simulink model "d01_Diaglnteg"  (R2024a)
settings: Solver=FixedStepDiscrete  StartTime=0.0  StopTime=1  FixedStep=mSim.dTime  MaxStep=Define.sModelSampleTime  RelTol=7.1420e-05
undefined symbols (not defined in the file): CnstMde, D01CRT, D01SPD, D01TEMP, D01VDC, D02DFLT
settings Model: Creator=user  LastModifiedBy=admin
settings SolverCC: MaxConsecutiveZCs=10000  ZeroCrossAlgorithm=Adaptive  AlgebraicLoopSolver=TrustRegion
settings DataIOCC: SaveOutput=off  DSMLogging=off  InspectSignalLogs=on  SaveTime=off  SignalLoggingName=logsout_Validator
settings OptimizationCC: BlockReduction=off  DefaultParameterBehavior=Inlined  UseDivisionForNetSlopeComputation=UseDivisionForReciprocalsOfIntegersOnly  GainParamInheritBuiltInType=on  UseFloatMulNetSlope=on  DefaultUnderspecifiedDataType=single  InlineInvariantSignals=on  BitwiseOrLogicalOp=Logical operator  PassReuseOutputArgsAs=Individual arguments  EfficientFloat2IntCast=on  LifeSpan=Inf  OptimizeBlockOrder=speed  DifferentSizesBufferReuse=on  EfficientTunableParamExpr=on
settings DebuggingCC: SignalInfNanChecking=error  SignalRangeChecking=error  ReadBeforeWriteMsg=EnableAllAsError  WriteAfterWriteMsg=EnableAllAsError  WriteAfterReadMsg=EnableAllAsError  AlgebraicLoopMsg=error  ArtificialAlgebraicLoopMsg=error  SaveWithDisabledLinksMsg=error  SaveWithParameterizedLinksMsg=error  BlockPriorityViolationMsg=error  SolverPrmCheckMsg=error  InheritedTsInSrcMsg=error  SingleTaskRateTransMsg=error  TasksWithSamePriorityMsg=error  SigSpecEnsureSampleTimeMsg=error  CheckMatrixSingularityMsg=error  IntegerOverflowMsg=error  ParameterUnderflowMsg=error  ParameterPrecisionLossMsg=error  ParameterTunabilityLossMsg=error  UnderSpecifiedDataTypeMsg=error  UnnecessaryDatatypeConvMsg=warning  VectorMatrixConversionMsg=error  SignalLabelMismatchMsg=error  UnconnectedInputMsg=error  UnconnectedOutputMsg=error  UnconnectedLineMsg=error  SFcnCompatibilityMsg=error  UniqueDataStoreMsg=error  BusObjectLabelMismatch=error  RootOutportRequireBusObject=error  AssertControl=DisableAll  ModelReferenceIOMismatchMessage=error  UnknownTsInhSupMsg=error  ModelReferenceDataLoggingMessage=error  ModelReferenceSymbolNameMessage=none  StateNameClashWarn=warning  StrictBusMsg=ErrorOnBusTreatedAsVector  NonBusSignalsTreatedAsBus=error  SFInvalidInputDataAccessInChartInitDiag=error  SFTransitionOutsideNaturalParentDiag=error  SFUnreachableExecutionPathDiag=error  SFUndirectedBroadcastEventsDiag=error  SFTransitionActionBeforeConditionDiag=error  SFTemporalDelaySmallerThanSampleTimeDiag=error  SFSelfTransitionDiag=error  SFExecutionAtInitializationDiag=error  IntegerSaturationMsg=error  UnitsInconsistencyMsg=none  VariantConditionMismatch=error
settings HardwareCC: ProdBitPerChar=16  ProdBitPerInt=16  ProdBitPerPointer=32  ProdBitPerSizeT=32  ProdBitPerPtrDiffT=32  ProdLargestAtomicInteger=Integer  ProdLargestAtomicFloat=None  ProdWordSize=16  ProdHWDeviceType=Texas Instruments->C2000
settings ModelReferenceCC: EnableRefExpFcnMdlSchedulingChecks=on  ModelReferenceNumInstancesAllowed=Single
settings SFSimCC: SimUseLocalCustomCode=off  CompileTimeRecursionLimit=0  EnableRuntimeRecursion=off  MATLABDynamicMemAlloc=off  CustomCodeUndefinedFunction=UseInterfaceOnly
settings RTWCC: Description=Embedded Coder  SystemTargetFile=ert.tlc  GenCodeOnly=on  TemplateMakefile=ert_default_tmf  GenerateReport=on  RTWUseLocalCustomCode=off  BuildConfiguration=Faster Runs  IncludeHyperlinkInReport=on  LaunchReport=on  GenerateTraceInfo=on  GenerateTraceReport=on  GenerateTraceReportSl=on  GenerateTraceReportSf=on  GenerateWebview=on  GenerateCodeMetricsReport=on  GenerateCodeReplacementReport=on  GPUComputeCapability=3.5  DLArmComputeVersion=19.05
settings CodeAppCC: ForceParamTrailComments=on  IgnoreCustomStorageClasses=off  MATLABFcnDesc=on  MangleLength=4  CustomSymbolStrGlobalVar=GvD01$N$M  CustomSymbolStrType=StrD01$N$M  CustomSymbolStrFcn=$N$M$F  CustomSymbolStrMacro=$N$M  DefineNamingRule=UpperCase  ParamNamingRule=UpperCase  SimulinkBlockComments=off  MATLABSourceComments=on  EnableCustomComments=on  ReqsInCode=on
settings ERTTargetCC: TargetLangStandard=C99 (ISO)  UtilityFuncGeneration=Shared location  MultiwordLength=2048  IncludeMdlTerminateFcn=off  CombineSignalStateStructs=on  SuppressErrorStatus=on  SupportAbsoluteTime=off  SupportNonFinite=off  ParenthesesLevel=Maximum  CastingMode=Standards  GenerateSharedConstants=off  InlinedParameterPlacement=NonHierarchical  ERTSrcFileBannerTemplate=t_code_template.cgt  ERTHdrFileBannerTemplate=t_code_template.cgt  ERTDataSrcFileTemplate=t_code_template.cgt  ERTDataHdrFileTemplate=t_code_template.cgt  ERTCustomFileTemplate=example_file_process.tlc  ERTFilePackagingFormat=CompactWithDataFile  PreserveExpressionOrder=on  SuppressUnreachableDefaultCases=off  EnableSignedLeftShifts=off  EnableSignedRightShifts=off  IndentStyle=Allman  IndentSize=4
settings ConfigComp: CovSaveName=coveragedata  CovMetricSettings=we  CovEnableCumulative=off  CovSaveCumulativeToWorkspaceVar=on  CovSaveSingleToWorkspaceVar=on  CovOutputDir=sldv_output/$ModelName$\sldv_covoutput  PSVerificationMode=BugFinder  PSModelRefIgnoreList=[]  PSEnableModelRefIgnoreList=off  PSModelRefMinMaxVerif=CheckAndConstrain  PSAutoStubLUT=on  DVModelCoverageObjectives=MCDC  DVTestSuiteOptimization=CombinedObjectives (Nonlinear Extended)  DVRebuildModelRepresentation=Always
settings SimscapeCC: SimscapeNormalizeSystem=off

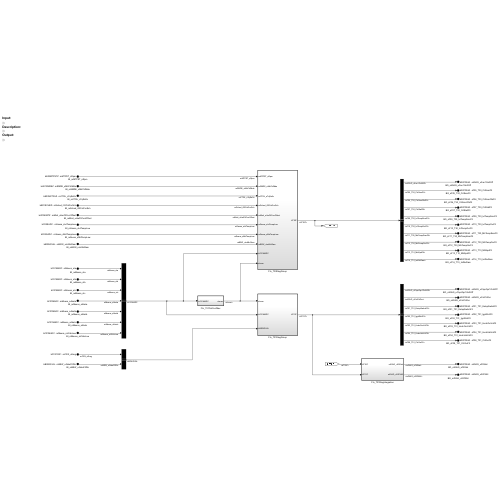
[thumbnail: Simulink's stored preview of the top-level diagram]
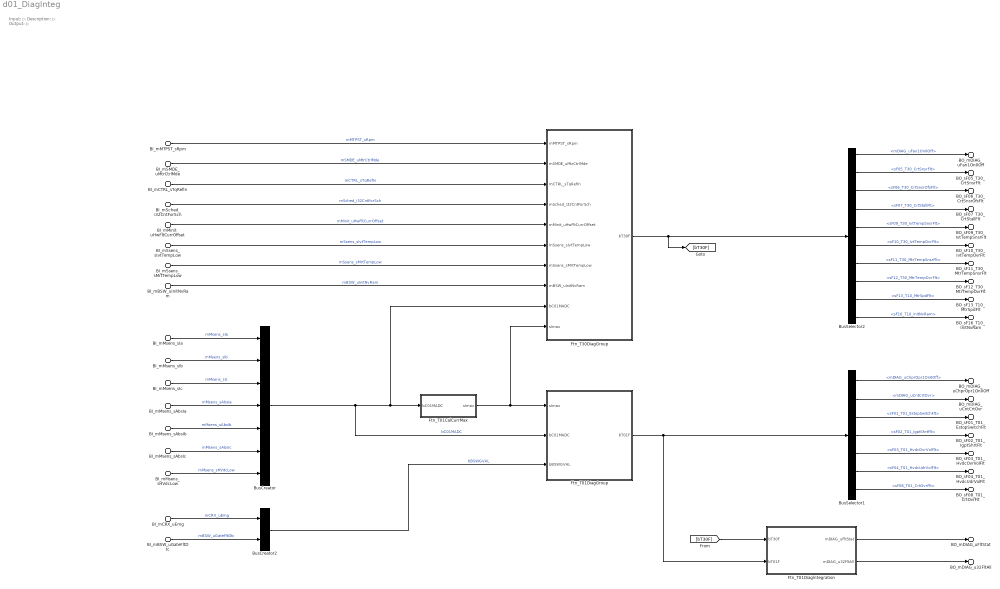
== system d01_Diaglnteg ==
  note: Input:
      | ▷
      | Description:
      | ▷
      | Output:
      | ▷
  BI_mMsens_sIa : Inport  PortName=bC01MADC  Element=mMsens_sIa
  BI_mMsens_sIb : Inport  PortName=bC01MADC  Element=mMsens_sIb
  BI_mMsens_sIc : Inport  PortName=bC01MADC  Element=mMsens_sIc
  BI_mMsens_sAbsIa : Inport  PortName=bC01MADC  Element=mMsens_sAbsIa
  BI_mMsens_sAbsIb : Inport  PortName=bC01MADC  Element=mMsens_sAbsIb
  BI_mMsens_sAbsIc : Inport  PortName=bC01MADC  Element=mMsens_sAbsIc
  BI_mMsens_sHVdcLow : Inport  PortName=bC01MADC  Element=mMsens_sHVdcLow
  BI_mSched_i32CntForSch : Inport  Port=2  PortName=bB01SCHED  Element=mSched_i32CntForSch
  BI_mMinit_uHwFltCurrOffset : Inport  Port=3  PortName=bJ01MINITZ  Element=mMinit_uHwFltCurrOffset
  BI_mCTRL_sTqRefIn : Inport  Port=4  PortName=bE03MCTRLZ  Element=mCTRL_sTqRefIn
  BI_mBSW_uGateFltDtc : Inport  Port=5  PortName=bBSWGVAL  Element=mBSW_uGateFltDtc
  BI_mBSW_uInitNvRam : Inport  Port=5  PortName=bBSWGVAL  Element=mBSW_uInitNvRam
  BI_mMTPST_sRpm : Inport  Port=6  PortName=bE02MTPSTZ  Element=mMTPST_sRpm
  BI_mSsens_sIvtTempLow : Inport  Port=7  PortName=bC02SADC  Element=mSsens_sIvtTempLow
  BI_mSsens_sMrtTempLow : Inport  Port=7  PortName=bC02SADC  Element=mSsens_sMrtTempLow
  BI_mSMDE_uMtrCtrlMde : Inport  Port=8  PortName=bH01SMDEZ  Element=mSMDE_uMtrCtrlMde
  BI_mCRX_uEmg : Inport  Description=■ 설명: Digital Input Signal (외부 비상 신호 입력, 0: 비상 신호 활성화, 1: 비상 신호 비활성화)  Port=9  PortName=bF01CRX1  Element=mCRX_uEmg
  BusCreator : BusCreator  Inputs=7
  BusCreator2 : BusCreator  Inputs=2
  BusSelector1 : BusSelector  OutputSignals=mDIAG_uChprOpr1On0Off,mDIAG_uCntCrtOvr,sF01_T01_EstopSwitchFlt,sF02_T01_IgptShrtFlt,sF03_T01_HvdcOvrVolFlt,sF04_T01_HvdcUdrVolFlt,sF08_T01_CrtOvrFlt
  BusSelector2 : BusSelector  OutputSignals=mDIAG_uFan1On0Off,sF05_T30_CrtSnsrFlt,sF06_T30_CrtSnsrOfsFlt,sF07_T30_CrtStallFlt,sF09_T30_IvtTempSnsrFlt,sF10_T30_IvtTempOvrFlt,sF11_T30_MtrTempSnsrFlt,sF12_T30_MtrTempOvrFlt,sF13_T10_MtrSpdFlt,sF16_T10_InitNvRam
  Ftn_T01CalCurrMax : Subsystem  TreatAsAtomicUnit=on
      settings: RTWSystemCode=Nonreusable function  RTWFcnNameOpts=Use subsystem name
  Ftn_T01DiagGroup : Subsystem  TreatAsAtomicUnit=on
      settings: RTWSystemCode=Nonreusable function  RTWFcnNameOpts=Use subsystem name
  Ftn_T01Diaglntegration : Subsystem  TreatAsAtomicUnit=on
      settings: RTWSystemCode=Nonreusable function  RTWFcnNameOpts=Use subsystem name
  Ftn_T30DiagGroup : Subsystem  TreatAsAtomicUnit=on
      settings: RTWSystemCode=Nonreusable function  RTWFcnNameOpts=Use subsystem name
  BO_mDIAG_uFltStat : Outport  Description=■ 설명: 고장 신호 대표 값  PortName=bD01DIAG  Element=mDIAG_uFltStat
  BO_mDIAG_u32FltAll : Outport  Description=■ 설명: 고장 신호 전체값  PortName=bD01DIAG  Element=mDIAG_u32FltAll
  BO_mDIAG_uChprOpr1On0Off : Outport  Description=■ 설명: Chopper 구동 신호 (0: Off, 1: On)  PortName=bD01DIAG  Element=mDIAG_uChprOpr1On0Off
  BO_mDIAG_uFan1On0Off : Outport  Description=■ 설명: Fan 구동 신호 (0: Off, 1: On)  PortName=bD01DIAG  Element=mDIAG_uFan1On0Off
  BO_mDIAG_uCntCrtOvr : Outport  Description=■ 설명: 과전류 검출 카운터  PortName=bD01DIAG  Element=mDIAG_uCntCrtOvr
  BO_sF01_T01_EstopSwitchFlt : Outport  Description=■ 설명: E-Stop Swhitch 검출 (0: Normal, 1: Fault)  PortName=bD01DIAG  Element=sF01_T01_EstopSwitchFlt
  BO_sF02_T01_IgptShrtFlt : Outport  Description=■ 설명: IGBT 고장 신호 (0: Normal, 1: Fault)  PortName=bD01DIAG  Element=sF02_T01_IgptShrtFlt
  BO_sF03_T01_HvdcOvrVolFlt : Outport  Description=■ 설명: DC Link 과전압 고장 검출 신호 (0: Normal, 1: Fault)  PortName=bD01DIAG  Element=sF03_T01_HvdcOvrVolFlt
  BO_sF04_T01_HvdcUdrVolFlt : Outport  Description=■ 설명: DC Link 저전압 고장 검출 신호 (0: Normal, 1: Fault)  PortName=bD01DIAG  Element=sF04_T01_HvdcUdrVolFlt
  BO_sF05_T30_CrtSnsrFlt : Outport  Description=■ 설명: 전류 센서 고장 검출 신호 (0: Normal, 1: Fault)  PortName=bD01DIAG  Element=sF05_T30_CrtSnsrFlt
  BO_sF06_T30_CrtSnsrOfsFlt : Outport  Description=■ 설명: 전류 센서 옵셋 고장 검출 신호 (0: Normal, 1: Fault)  PortName=bD01DIAG  Element=sF06_T30_CrtSnsrOfsFlt
  BO_sF07_T30_CrtStallFlt : Outport  Description=■ 설명: 구속 전류 고장 검출 신호 (0: Normal, 1: Fault)  PortName=bD01DIAG  Element=sF07_T30_CrtStallFlt
  BO_sF08_T01_CrtOvrFlt : Outport  Description=■ 설명: 과전류 고장 검출 신호 (0: Normal, 1: Fault)  PortName=bD01DIAG  Element=sF08_T01_CrtOvrFlt
  BO_sF09_T30_IvtTempSnsrFlt : Outport  Description=■ 설명: IGBT 온도 센서 고장 검출 신호 (0: Normal, 1: Fault)  PortName=bD01DIAG  Element=sF09_T30_IvtTempSnsrFlt
  BO_sF10_T30_IvtTempOvrFlt : Outport  Description=■ 설명: IGBT 과온 고장 검출 신호 (0: Normal, 1: Fault)  PortName=bD01DIAG  Element=sF10_T30_IvtTempOvrFlt
  BO_sF11_T30_MtrTempSnsrFlt : Outport  Description=■ 설명: 모터 온도 센서 고장 검출 신호 (0: Normal, 1: Fault)  PortName=bD01DIAG  Element=sF11_T30_MtrTempSnsrFlt
  BO_sF12_T30_MtrTempOvrFlt : Outport  Description=■ 설명: 모터 과온 고장 검출 신호 (0: Normal, 1: Fault)  PortName=bD01DIAG  Element=sF12_T30_MtrTempOvrFlt
  BO_sF13_T10_MtrSpdFlt : Outport  Description="■ 설명: 과속 고장 검출 신호  (0: Normal, 1: Fault)"  PortName=bD01DIAG  Element=sF13_T10_MtrSpdFlt
  BO_sF16_T10_InitNvRam : Outport  Description=■ 설명: 모터 과온 고장 검출 신호 (0: Normal, 1: Fault)  PortName=bD01DIAG  Element=sF16_T10_InitNvRam
  wires:
  BI_mMsens_sIa/1 -> BusCreator/1  "mMsens_sIa"
  BI_mMsens_sIb/1 -> BusCreator/2  "mMsens_sIb"
  BI_mMsens_sIc/1 -> BusCreator/3  "mMsens_sIc"
  BI_mMsens_sAbsIa/1 -> BusCreator/4  "mMsens_sAbsIa"
  BI_mMsens_sAbsIb/1 -> BusCreator/5  "mMsens_sAbsIb"
  BI_mMsens_sAbsIc/1 -> BusCreator/6  "mMsens_sAbsIc"
  BI_mMsens_sHVdcLow/1 -> BusCreator/7  "mMsens_sHVdcLow"
  BusCreator/1 -> Ftn_T01CalCurrMax/1(bC01MADC), Ftn_T30DiagGroup/9(bC01MADC), Ftn_T01DiagGroup/2(bC01MADC)  "bC01MADC"
  Ftn_T01CalCurrMax/1(sImax) -> Ftn_T30DiagGroup/10(sImax), Ftn_T01DiagGroup/1(sImax)
  Ftn_T01DiagGroup/1(bT01F) -> BusSelector1/1, Ftn_T01Diaglntegration/2(bT01F)
  BusSelector1/1 -> BO_mDIAG_uChprOpr1On0Off/1  "<mDIAG_uChprOpr1On0Off>"
  BusSelector1/5 -> BO_sF03_T01_HvdcOvrVolFlt/1  "<sF03_T01_HvdcOvrVolFlt>"
  BusSelector1/6 -> BO_sF04_T01_HvdcUdrVolFlt/1  "<sF04_T01_HvdcUdrVolFlt>"
  BI_mSched_i32CntForSch/1 -> Ftn_T30DiagGroup/4(mSched_i32CntForSch)  "mSched_i32CntForSch"
  BusSelector1/7 -> BO_sF08_T01_CrtOvrFlt/1  "<sF08_T01_CrtOvrFlt>"
  BusSelector1/2 -> BO_mDIAG_uCntCrtOvr/1  "<mDIAG_uCntCrtOvr>"
  BI_mMinit_uHwFltCurrOffset/1 -> Ftn_T30DiagGroup/5(mMinit_uHwFltCurrOffset)  "mMinit_uHwFltCurrOffset"
  BI_mSMDE_uMtrCtrlMde/1 -> Ftn_T30DiagGroup/2(mSMDE_uMtrCtrlMde)  "mSMDE_uMtrCtrlMde"
  BI_mCTRL_sTqRefIn/1 -> Ftn_T30DiagGroup/3(mCTRL_sTqRefIn)  "mCTRL_sTqRefIn"
  Ftn_T30DiagGroup/1(bT30F) -> [bT30F], BusSelector2/1
  BusSelector2/2 -> BO_sF05_T30_CrtSnsrFlt/1  "<sF05_T30_CrtSnsrFlt>"
  BusSelector2/3 -> BO_sF06_T30_CrtSnsrOfsFlt/1  "<sF06_T30_CrtSnsrOfsFlt>"
  BusSelector2/4 -> BO_sF07_T30_CrtStallFlt/1  "<sF07_T30_CrtStallFlt>"
  BI_mBSW_uGateFltDtc/1 -> BusCreator2/2  "mBSW_uGateFltDtc"
  BusCreator2/1 -> Ftn_T01DiagGroup/3(bBSWGVAL)  "bBSWGVAL"
  BusSelector1/3 -> BO_sF01_T01_EstopSwitchFlt/1  "<sF01_T01_EstopSwitchFlt>"
  BusSelector1/4 -> BO_sF02_T01_IgptShrtFlt/1  "<sF02_T01_IgptShrtFlt>"
  BI_mMTPST_sRpm/1 -> Ftn_T30DiagGroup/1(mMTPST_sRpm)  "mMTPST_sRpm"
  BusSelector2/9 -> BO_sF13_T10_MtrSpdFlt/1  "<sF13_T10_MtrSpdFlt>"
  BI_mSsens_sIvtTempLow/1 -> Ftn_T30DiagGroup/6(mSsens_sIvtTempLow)  "mSsens_sIvtTempLow"
  BI_mSsens_sMrtTempLow/1 -> Ftn_T30DiagGroup/7(mSsens_sMrtTempLow)  "mSsens_sMrtTempLow"
  BusSelector2/5 -> BO_sF09_T30_IvtTempSnsrFlt/1  "<sF09_T30_IvtTempSnsrFlt>"
  BusSelector2/6 -> BO_sF10_T30_IvtTempOvrFlt/1  "<sF10_T30_IvtTempOvrFlt>"
  BusSelector2/7 -> BO_sF11_T30_MtrTempSnsrFlt/1  "<sF11_T30_MtrTempSnsrFlt>"
  BusSelector2/8 -> BO_sF12_T30_MtrTempOvrFlt/1  "<sF12_T30_MtrTempOvrFlt>"
  BusSelector2/1 -> BO_mDIAG_uFan1On0Off/1  "<mDIAG_uFan1On0Off>"
  [bT30F] -> Ftn_T01Diaglntegration/1(bT30F)
  Ftn_T01Diaglntegration/2(mDIAG_u32FltAll) -> BO_mDIAG_u32FltAll/1
  Ftn_T01Diaglntegration/1(mDIAG_uFltStat) -> BO_mDIAG_uFltStat/1
  BI_mBSW_uInitNvRam/1 -> Ftn_T30DiagGroup/8(mBSW_uInitNvRam)  "mBSW_uInitNvRam"
  BusSelector2/10 -> BO_sF16_T10_InitNvRam/1  "<sF16_T10_InitNvRam>"
  BI_mCRX_uEmg/1 -> BusCreator2/1  "mCRX_uEmg"

== system d01_Diaglnteg/Ftn_T01CalCurrMax ==
  note: Input:
      | Description:
      | Output:
  bC01MADC : Inport
  BusSelector : BusSelector  OutputSignals=mMsens_sAbsIa,mMsens_sAbsIb,mMsens_sAbsIc
  Max : MinMax  Function=max  Inputs=3
  sImax : Outport
  wires:
  Max/1 -> sImax/1  "sImax"
  bC01MADC/1 -> BusSelector/1
  BusSelector/2 -> Max/2  "<mMsens_sAbsIb>"
  BusSelector/1 -> Max/1  "<mMsens_sAbsIa>"
  BusSelector/3 -> Max/3  "<mMsens_sAbsIc>"

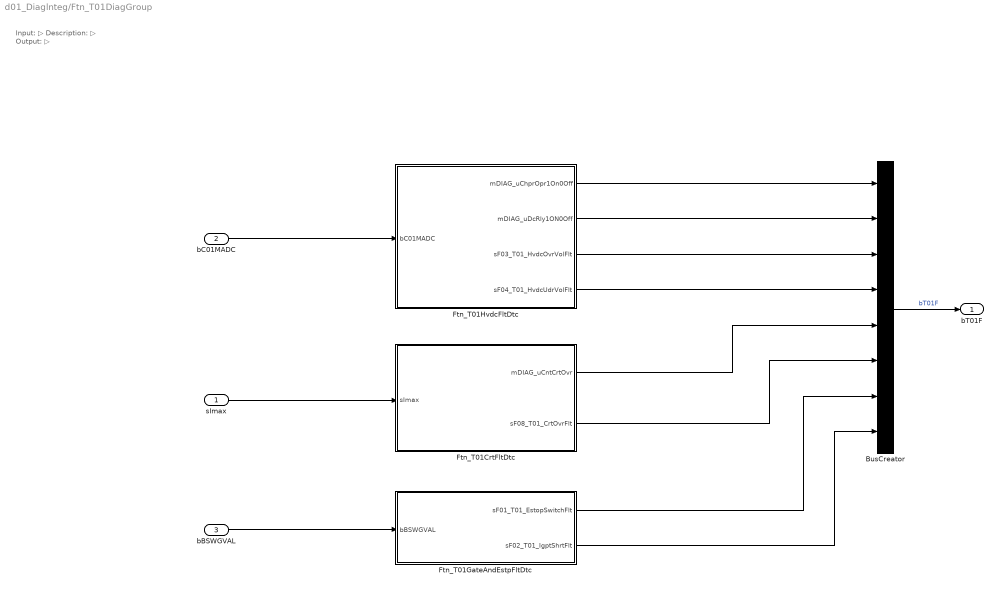
== system d01_Diaglnteg/Ftn_T01DiagGroup ==
  note: Input:
      | ▷
      | Description:
      | ▷
      | Output:
      | ▷
  sImax : Inport
  bC01MADC : Inport  Port=2
  bBSWGVAL : Inport  Port=3
  BusCreator : BusCreator  Inputs=8
  Ftn_T01CrtFltDtc : Subsystem  TreatAsAtomicUnit=on
      settings: RTWSystemCode=Nonreusable function  RTWFcnNameOpts=Use subsystem name
  Ftn_T01GateAndEstpFltDtc : Subsystem  TreatAsAtomicUnit=on
      settings: RTWSystemCode=Nonreusable function  RTWFcnNameOpts=Use subsystem name
  Ftn_T01HvdcFltDtc : Subsystem  TreatAsAtomicUnit=on
      settings: RTWSystemCode=Nonreusable function  RTWFcnNameOpts=Use subsystem name
  bT01F : Outport
  wires:
  bC01MADC/1 -> Ftn_T01HvdcFltDtc/1(bC01MADC)
  sImax/1 -> Ftn_T01CrtFltDtc/1(sImax)
  Ftn_T01HvdcFltDtc/1(mDIAG_uChprOpr1On0Off) -> BusCreator/1
  Ftn_T01HvdcFltDtc/3(sF03_T01_HvdcOvrVolFlt) -> BusCreator/3
  Ftn_T01HvdcFltDtc/4(sF04_T01_HvdcUdrVolFlt) -> BusCreator/4
  BusCreator/1 -> bT01F/1  "bT01F"
  Ftn_T01CrtFltDtc/1(mDIAG_uCntCrtOvr) -> BusCreator/5
  Ftn_T01CrtFltDtc/2(sF08_T01_CrtOvrFlt) -> BusCreator/6
  Ftn_T01GateAndEstpFltDtc/1(sF01_T01_EstopSwitchFlt) -> BusCreator/7
  bBSWGVAL/1 -> Ftn_T01GateAndEstpFltDtc/1(bBSWGVAL)
  Ftn_T01GateAndEstpFltDtc/2(sF02_T01_IgptShrtFlt) -> BusCreator/8
  Ftn_T01HvdcFltDtc/2(mDIAG_uDcRly1ON0Off) -> BusCreator/2

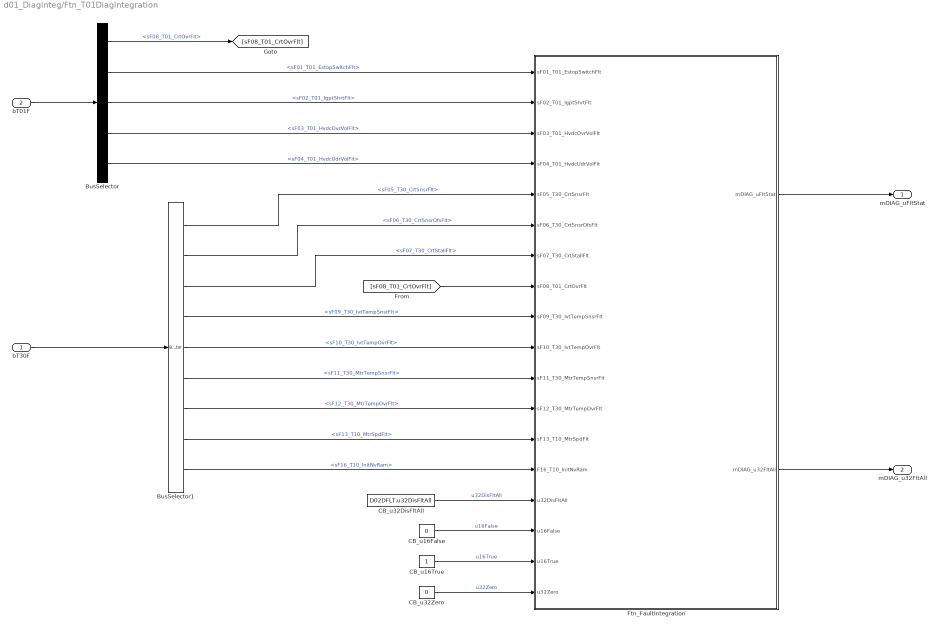
== system d01_Diaglnteg/Ftn_T01Diaglntegration ==
  bT30F : Inport
  bT01F : Inport  Port=2
  BusSelector : BusSelector  OutputSignals=sF08_T01_CrtOvrFlt,sF01_T01_EstopSwitchFlt,sF02_T01_IgptShrtFlt,sF03_T01_HvdcOvrVolFlt,sF04_T01_HvdcUdrVolFlt
  BusSelector1 : BusSelector  OutputSignals=sF05_T30_CrtSnsrFlt,sF06_T30_CrtSnsrOfsFlt,sF07_T30_CrtStallFlt,sF09_T30_IvtTempSnsrFlt,sF10_T30_IvtTempOvrFlt,sF11_T30_MtrTempSnsrFlt,sF12_T30_MtrTempOvrFlt,sF13_T10_MtrSpdFlt,sF16_T10_InitNvRam
  CB_u16False : Constant  Value=0  OutDataTypeStr=uint16
  CB_u16True : Constant  OutDataTypeStr=uint16
  CB_u32DisFltAll : Constant  Value=D02DFLT.u32DisFltAll
  CB_u32Zero : Constant  Value=0  OutDataTypeStr=uint32
  Ftn_FaultIntegration : Stateflow chart  TreatAsAtomicUnit=on
      settings: RTWSystemCode=Nonreusable function
  mDIAG_uFltStat : Outport
  mDIAG_u32FltAll : Outport  Port=2
  wires:
  bT01F/1 -> BusSelector/1
  BusSelector/2 -> Ftn_FaultIntegration/1(sF01_T01_EstopSwitchFlt)  "<sF01_T01_EstopSwitchFlt>"
  BusSelector/3 -> Ftn_FaultIntegration/2(sF02_T01_IgptShrtFlt)  "<sF02_T01_IgptShrtFlt>"
  BusSelector/1 -> [sF08_T01_CrtOvrFlt]  "<sF08_T01_CrtOvrFlt>"
  bT30F/1 -> BusSelector1/1
  BusSelector1/2 -> Ftn_FaultIntegration/6(sF06_T30_CrtSnsrOfsFlt)  "<sF06_T30_CrtSnsrOfsFlt>"
  BusSelector1/3 -> Ftn_FaultIntegration/7(sF07_T30_CrtStallFlt)  "<sF07_T30_CrtStallFlt>"
  BusSelector1/4 -> Ftn_FaultIntegration/9(sF09_T30_IvtTempSnsrFlt)  "<sF09_T30_IvtTempSnsrFlt>"
  BusSelector1/5 -> Ftn_FaultIntegration/10(sF10_T30_IvtTempOvrFlt)  "<sF10_T30_IvtTempOvrFlt>"
  BusSelector1/6 -> Ftn_FaultIntegration/11(sF11_T30_MtrTempSnsrFlt)  "<sF11_T30_MtrTempSnsrFlt>"
  BusSelector1/7 -> Ftn_FaultIntegration/12(sF12_T30_MtrTempOvrFlt)  "<sF12_T30_MtrTempOvrFlt>"
  BusSelector1/8 -> Ftn_FaultIntegration/13(sF13_T10_MtrSpdFlt)  "<sF13_T10_MtrSpdFlt>"
  BusSelector/4 -> Ftn_FaultIntegration/3(sF03_T01_HvdcOvrVolFlt)  "<sF03_T01_HvdcOvrVolFlt>"
  BusSelector/5 -> Ftn_FaultIntegration/4(sF04_T01_HvdcUdrVolFlt)  "<sF04_T01_HvdcUdrVolFlt>"
  BusSelector1/1 -> Ftn_FaultIntegration/5(sF05_T30_CrtSnsrFlt)  "<sF05_T30_CrtSnsrFlt>"
  [sF08_T01_CrtOvrFlt] -> Ftn_FaultIntegration/8(sF08_T01_CrtOvrFlt)
  CB_u32DisFltAll/1 -> Ftn_FaultIntegration/15(u32DisFltAll)  "u32DisFltAll"
  CB_u16False/1 -> Ftn_FaultIntegration/16(u16False)  "u16False"
  CB_u16True/1 -> Ftn_FaultIntegration/17(u16True)  "u16True"
  CB_u32Zero/1 -> Ftn_FaultIntegration/18(u32Zero)  "u32Zero"
  Ftn_FaultIntegration/1(mDIAG_uFltStat) -> mDIAG_uFltStat/1
  Ftn_FaultIntegration/2(mDIAG_u32FltAll) -> mDIAG_u32FltAll/1
  BusSelector1/9 -> Ftn_FaultIntegration/14(F16_T10_InitNvRam)  "<sF16_T10_InitNvRam>"

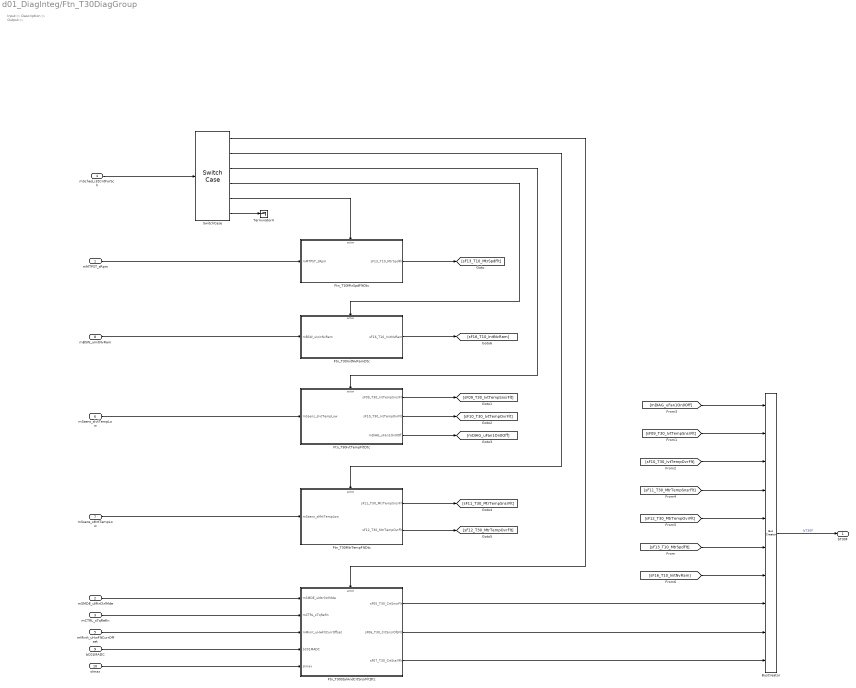
== system d01_Diaglnteg/Ftn_T30DiagGroup ==
  note: Input:
      | ▷
      | Description:
      | ▷
      | Output:
      | ▷
  mMTPST_sRpm : Inport
  mSMDE_uMtrCtrlMde : Inport  Port=2
  mCTRL_sTqRefIn : Inport  Port=3
  mSched_i32CntForSch : Inport  Port=4
  mMinit_uHwFltCurrOffset : Inport  Port=5
  mSsens_sIvtTempLow : Inport  Port=6
  mSsens_sMrtTempLow : Inport  Port=7
  mBSW_uInitNvRam : Inport  Port=8
  bC01MADC : Inport  Port=9
  sImax : Inport  Port=10
  BusCreator : BusCreator  Inputs=10
  Ftn_T10MtrSpdFltDtc : Subsystem  TreatAsAtomicUnit=on
      settings: RTWSystemCode=Nonreusable function  RTWFcnNameOpts=Use subsystem name
  Ftn_T30InitNvRamDtc : Subsystem
      settings: RTWSystemCode=Nonreusable function  RTWFcnNameOpts=Use subsystem name
  Ftn_T30IvtTempFltDtc : Subsystem  TreatAsAtomicUnit=on
      settings: RTWSystemCode=Nonreusable function  RTWFcnNameOpts=Use subsystem name
  Ftn_T30MtrTempFltDtc : Subsystem  TreatAsAtomicUnit=on
      settings: RTWSystemCode=Nonreusable function  RTWFcnNameOpts=Use subsystem name
  Ftn_T30StalAndCrtSnsrFltDtc : Subsystem  TreatAsAtomicUnit=on
      settings: RTWSystemCode=Nonreusable function  RTWFcnNameOpts=Use subsystem name
  SwitchCase : SwitchCase  CaseConditions={28, 24,18, 2, [6,26]}
  Terminator4 : Terminator
  bT30F : Outport
  wires:
  SwitchCase/6 -> Terminator4/1
  mSched_i32CntForSch/1 -> SwitchCase/1
  mMinit_uHwFltCurrOffset/1 -> Ftn_T30StalAndCrtSnsrFltDtc/3(mMinit_uHwFltCurrOffset)
  bC01MADC/1 -> Ftn_T30StalAndCrtSnsrFltDtc/4(bC01MADC)
  sImax/1 -> Ftn_T30StalAndCrtSnsrFltDtc/5(sImax)
  mCTRL_sTqRefIn/1 -> Ftn_T30StalAndCrtSnsrFltDtc/2(mCTRL_sTqRefIn)
  mSMDE_uMtrCtrlMde/1 -> Ftn_T30StalAndCrtSnsrFltDtc/1(mSMDE_uMtrCtrlMde)
  Ftn_T30StalAndCrtSnsrFltDtc/1(sF05_T30_CrtSnsrFlt) -> BusCreator/8
  Ftn_T30StalAndCrtSnsrFltDtc/2(sF06_T30_CrtSnsrOfsFlt) -> BusCreator/9
  Ftn_T30StalAndCrtSnsrFltDtc/3(sF07_T30_CrtStallFlt) -> BusCreator/10
  BusCreator/1 -> bT30F/1  "bT30F"
  SwitchCase/1 -> Ftn_T30StalAndCrtSnsrFltDtc/Action
  SwitchCase/4 -> Ftn_T30InitNvRamDtc/Action
  mMTPST_sRpm/1 -> Ftn_T10MtrSpdFltDtc/1(mMTPST_sRpm)
  Ftn_T10MtrSpdFltDtc/1(sF13_T10_MtrSpdFlt) -> [sF13_T10_MtrSpdFlt]
  [sF13_T10_MtrSpdFlt] -> BusCreator/6
  SwitchCase/3 -> Ftn_T30IvtTempFltDtc/Action
  mSsens_sIvtTempLow/1 -> Ftn_T30IvtTempFltDtc/1(mSsens_sIvtTempLow)
  Ftn_T30IvtTempFltDtc/1(sF09_T30_IvtTempSnsrFlt) -> [sF09_T30_IvtTempSnsrFlt]
  Ftn_T30IvtTempFltDtc/2(sF10_T30_IvtTempOvrFlt) -> [sF10_T30_IvtTempOvrFlt]
  Ftn_T30IvtTempFltDtc/3(mDIAG_uFan1On0Off) -> [mDIAG_uFan1On0Off]
  [sF09_T30_IvtTempSnsrFlt] -> BusCreator/2
  [sF10_T30_IvtTempOvrFlt] -> BusCreator/3
  [mDIAG_uFan1On0Off] -> BusCreator/1
  mSsens_sMrtTempLow/1 -> Ftn_T30MtrTempFltDtc/1(mSsens_sMrtTempLow)
  Ftn_T30MtrTempFltDtc/1(sF11_T30_MtrTempSnsrFlt) -> [sF11_T30_MtrTempSnsrFlt]
  Ftn_T30MtrTempFltDtc/2(sF12_T30_MtrTempOvrFlt) -> [sF12_T30_MtrTempOvrFlt]
  [sF11_T30_MtrTempSnsrFlt] -> BusCreator/4
  [sF12_T30_MtrTempOvrFlt] -> BusCreator/5
  SwitchCase/2 -> Ftn_T30MtrTempFltDtc/Action
  mBSW_uInitNvRam/1 -> Ftn_T30InitNvRamDtc/1(mBSW_uInitNvRam)
  Ftn_T30InitNvRamDtc/1(sF16_T10_InitNvRam) -> [sF16_T10_InitNvRam]
  [sF16_T10_InitNvRam] -> BusCreator/7
  SwitchCase/5 -> Ftn_T10MtrSpdFltDtc/Action

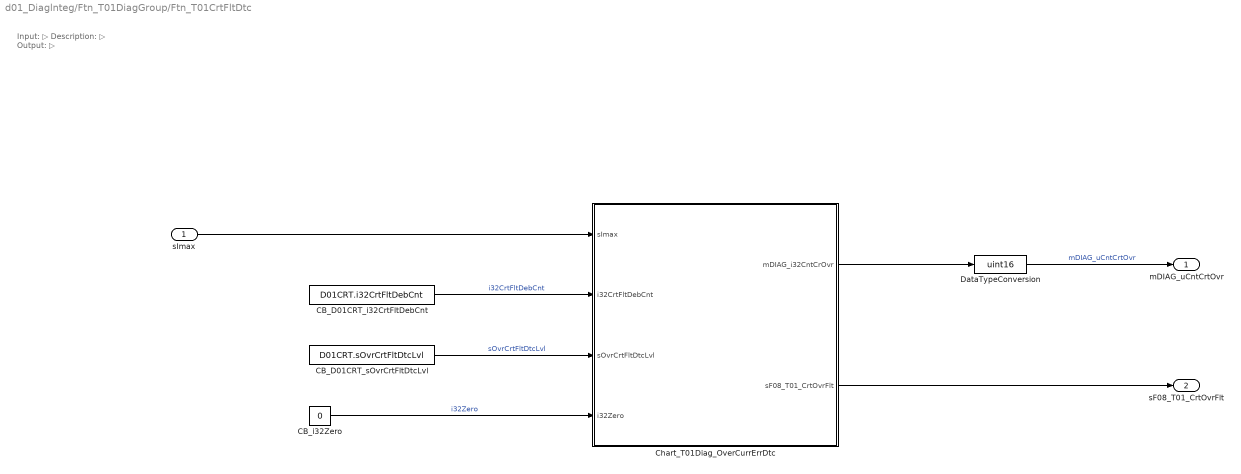
== system d01_Diaglnteg/Ftn_T01DiagGroup/Ftn_T01CrtFltDtc ==
  note: Input:
      | ▷
      | Description:
      | ▷
      | Output:
      | ▷
  sImax : Inport
  CB_D01CRT_i32CrtFltDebCnt : Constant  Value=D01CRT.i32CrtFltDebCnt
  CB_D01CRT_sOvrCrtFltDtcLvl : Constant  Value=D01CRT.sOvrCrtFltDtcLvl
  CB_i32Zero : Constant  Value=0  OutDataTypeStr=int32
  Chart_T01Diag_OverCurrErrDtc : Stateflow chart  TreatAsAtomicUnit=on
  DataTypeConversion : DataTypeConversion  OutDataTypeStr=uint16  SaturateOnIntegerOverflow=off  RndMeth=Floor
  mDIAG_uCntCrtOvr : Outport
  sF08_T01_CrtOvrFlt : Outport  Port=2
  wires:
  DataTypeConversion/1 -> mDIAG_uCntCrtOvr/1  "mDIAG_uCntCrtOvr"
  CB_i32Zero/1 -> Chart_T01Diag_OverCurrErrDtc/4(i32Zero)  "i32Zero"
  Chart_T01Diag_OverCurrErrDtc/1(mDIAG_i32CntCrOvr) -> DataTypeConversion/1
  Chart_T01Diag_OverCurrErrDtc/2(sF08_T01_CrtOvrFlt) -> sF08_T01_CrtOvrFlt/1
  CB_D01CRT_sOvrCrtFltDtcLvl/1 -> Chart_T01Diag_OverCurrErrDtc/3(sOvrCrtFltDtcLvl)  "sOvrCrtFltDtcLvl"
  CB_D01CRT_i32CrtFltDebCnt/1 -> Chart_T01Diag_OverCurrErrDtc/2(i32CrtFltDebCnt)  "i32CrtFltDebCnt"
  sImax/1 -> Chart_T01Diag_OverCurrErrDtc/1(sImax)

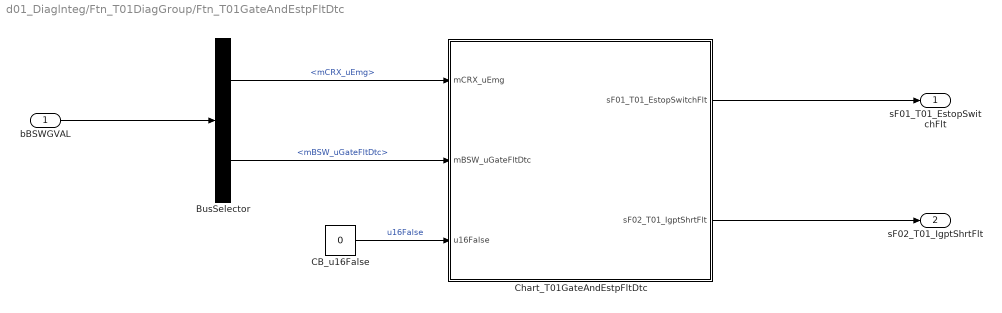
== system d01_Diaglnteg/Ftn_T01DiagGroup/Ftn_T01GateAndEstpFltDtc ==
  bBSWGVAL : Inport
  BusSelector : BusSelector  OutputSignals=mCRX_uEmg,mBSW_uGateFltDtc
  CB_u16False : Constant  Value=0  OutDataTypeStr=uint16
  Chart_T01GateAndEstpFltDtc : Stateflow chart  TreatAsAtomicUnit=on
  sF01_T01_EstopSwitchFlt : Outport
  sF02_T01_IgptShrtFlt : Outport  Port=2
  wires:
  bBSWGVAL/1 -> BusSelector/1
  BusSelector/1 -> Chart_T01GateAndEstpFltDtc/1(mCRX_uEmg)  "<mCRX_uEmg>"
  BusSelector/2 -> Chart_T01GateAndEstpFltDtc/2(mBSW_uGateFltDtc)  "<mBSW_uGateFltDtc>"
  Chart_T01GateAndEstpFltDtc/1(sF01_T01_EstopSwitchFlt) -> sF01_T01_EstopSwitchFlt/1
  Chart_T01GateAndEstpFltDtc/2(sF02_T01_IgptShrtFlt) -> sF02_T01_IgptShrtFlt/1
  CB_u16False/1 -> Chart_T01GateAndEstpFltDtc/3(u16False)  "u16False"

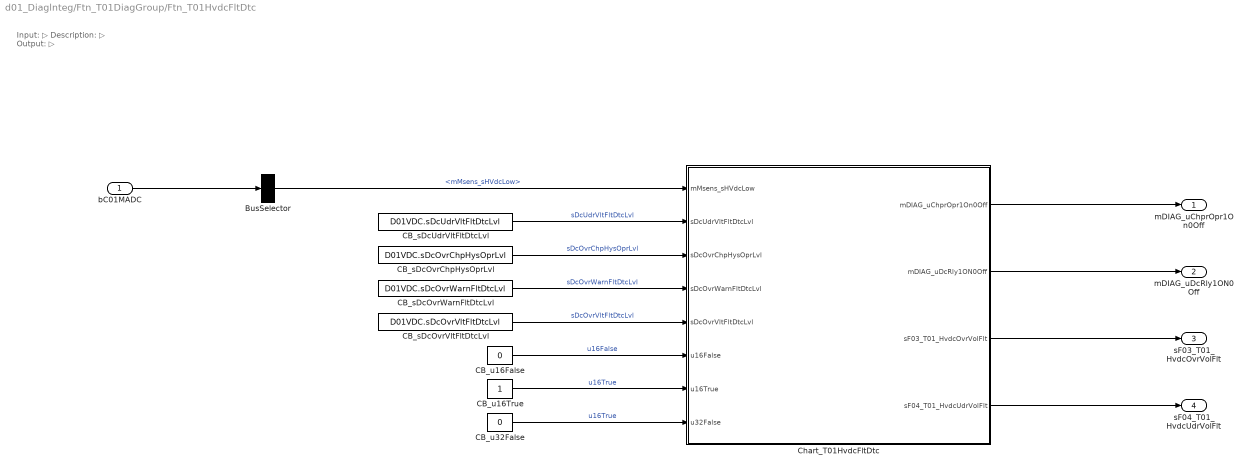
== system d01_Diaglnteg/Ftn_T01DiagGroup/Ftn_T01HvdcFltDtc ==
  note: Input:
      | ▷
      | Description:
      | ▷
      | Output:
      | ▷
  bC01MADC : Inport
  BusSelector : BusSelector  OutputSignals=mMsens_sHVdcLow
  CB_sDcOvrChpHysOprLvl : Constant  Value=D01VDC.sDcOvrChpHysOprLvl
  CB_sDcOvrVltFltDtcLvl : Constant  Value=D01VDC.sDcOvrVltFltDtcLvl
  CB_sDcOvrWarnFltDtcLvl : Constant  Value=D01VDC.sDcOvrWarnFltDtcLvl
  CB_sDcUdrVltFltDtcLvl : Constant  Value=D01VDC.sDcUdrVltFltDtcLvl
  CB_u16False : Constant  Value=0  OutDataTypeStr=uint16
  CB_u16True : Constant  OutDataTypeStr=uint16
  CB_u32False : Constant  Value=0  OutDataTypeStr=uint32
  Chart_T01HvdcFltDtc : Stateflow chart  TreatAsAtomicUnit=on
  mDIAG_uChprOpr1On0Off : Outport
  mDIAG_uDcRly1ON0Off : Outport  Port=2
  sF03_T01_HvdcOvrVolFlt : Outport  Port=3
  sF04_T01_HvdcUdrVolFlt : Outport  Port=4
  wires:
  bC01MADC/1 -> BusSelector/1
  BusSelector/1 -> Chart_T01HvdcFltDtc/1(mMsens_sHVdcLow)  "<mMsens_sHVdcLow>"
  CB_sDcUdrVltFltDtcLvl/1 -> Chart_T01HvdcFltDtc/2(sDcUdrVltFltDtcLvl)  "sDcUdrVltFltDtcLvl"
  CB_sDcOvrChpHysOprLvl/1 -> Chart_T01HvdcFltDtc/3(sDcOvrChpHysOprLvl)  "sDcOvrChpHysOprLvl"
  CB_sDcOvrWarnFltDtcLvl/1 -> Chart_T01HvdcFltDtc/4(sDcOvrWarnFltDtcLvl)  "sDcOvrWarnFltDtcLvl"
  CB_sDcOvrVltFltDtcLvl/1 -> Chart_T01HvdcFltDtc/5(sDcOvrVltFltDtcLvl)  "sDcOvrVltFltDtcLvl"
  CB_u16False/1 -> Chart_T01HvdcFltDtc/6(u16False)  "u16False"
  CB_u16True/1 -> Chart_T01HvdcFltDtc/7(u16True)  "u16True"
  Chart_T01HvdcFltDtc/1(mDIAG_uChprOpr1On0Off) -> mDIAG_uChprOpr1On0Off/1
  Chart_T01HvdcFltDtc/3(sF03_T01_HvdcOvrVolFlt) -> sF03_T01_HvdcOvrVolFlt/1
  Chart_T01HvdcFltDtc/4(sF04_T01_HvdcUdrVolFlt) -> sF04_T01_HvdcUdrVolFlt/1
  Chart_T01HvdcFltDtc/2(mDIAG_uDcRly1ON0Off) -> mDIAG_uDcRly1ON0Off/1
  CB_u32False/1 -> Chart_T01HvdcFltDtc/8(u32False)  "u16True"

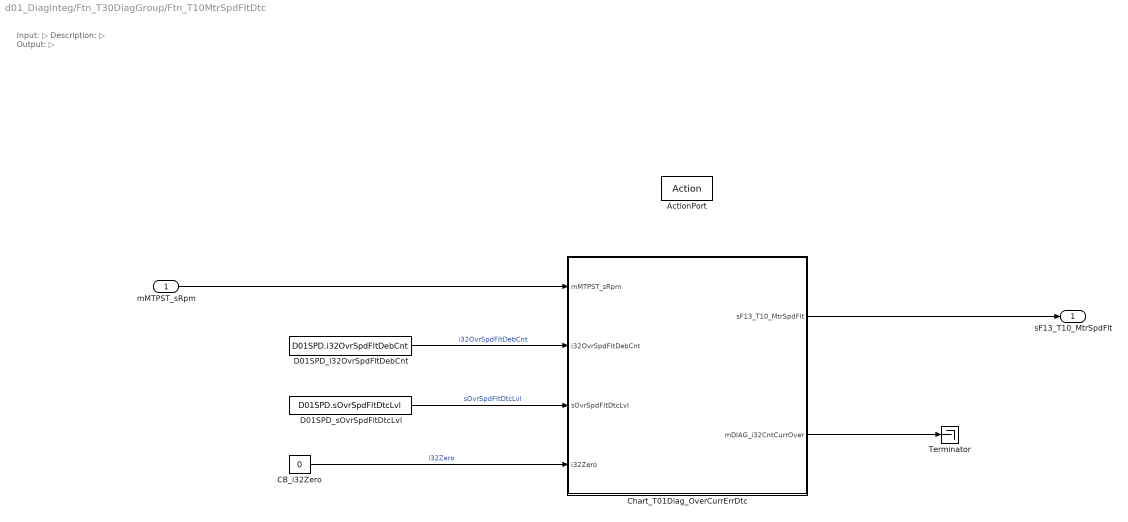
== system d01_Diaglnteg/Ftn_T30DiagGroup/Ftn_T10MtrSpdFltDtc ==
  note: Input:
      | ▷
      | Description:
      | ▷
      | Output:
      | ▷
  mMTPST_sRpm : Inport
  ActionPort : ActionPort  ActionPortLabel=case [ 6 26 ]:
  CB_i32Zero : Constant  Value=0  OutDataTypeStr=int32
  Chart_T01Diag_OverCurrErrDtc : Stateflow chart  TreatAsAtomicUnit=on
  D01SPD_i32OvrSpdFltDebCnt : Constant  Value=D01SPD.i32OvrSpdFltDebCnt
  D01SPD_sOvrSpdFltDtcLvl : Constant  Value=D01SPD.sOvrSpdFltDtcLvl
  Terminator : Terminator
  sF13_T10_MtrSpdFlt : Outport
  wires:
  D01SPD_sOvrSpdFltDtcLvl/1 -> Chart_T01Diag_OverCurrErrDtc/3(sOvrSpdFltDtcLvl)  "sOvrSpdFltDtcLvl"
  Chart_T01Diag_OverCurrErrDtc/1(sF13_T10_MtrSpdFlt) -> sF13_T10_MtrSpdFlt/1
  D01SPD_i32OvrSpdFltDebCnt/1 -> Chart_T01Diag_OverCurrErrDtc/2(i32OvrSpdFltDebCnt)  "i32OvrSpdFltDebCnt"
  CB_i32Zero/1 -> Chart_T01Diag_OverCurrErrDtc/4(i32Zero)  "i32Zero"
  Chart_T01Diag_OverCurrErrDtc/2(mDIAG_i32CntCurrOver) -> Terminator/1
  mMTPST_sRpm/1 -> Chart_T01Diag_OverCurrErrDtc/1(mMTPST_sRpm)

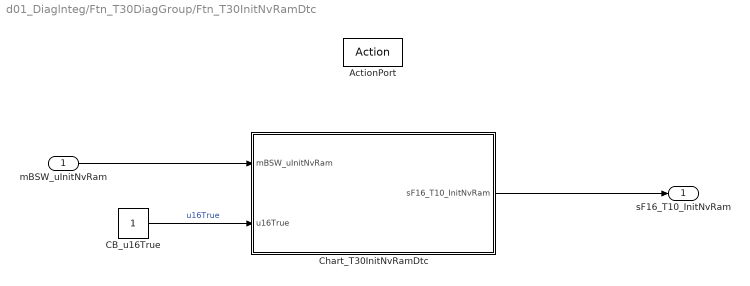
== system d01_Diaglnteg/Ftn_T30DiagGroup/Ftn_T30InitNvRamDtc ==
  mBSW_uInitNvRam : Inport
  ActionPort : ActionPort  ActionPortLabel=case [ 2 ]:
  CB_u16True : Constant  OutDataTypeStr=uint16
  Chart_T30InitNvRamDtc : Stateflow chart  TreatAsAtomicUnit=on
  sF16_T10_InitNvRam : Outport
  wires:
  CB_u16True/1 -> Chart_T30InitNvRamDtc/2(u16True)  "u16True"
  mBSW_uInitNvRam/1 -> Chart_T30InitNvRamDtc/1(mBSW_uInitNvRam)
  Chart_T30InitNvRamDtc/1(sF16_T10_InitNvRam) -> sF16_T10_InitNvRam/1

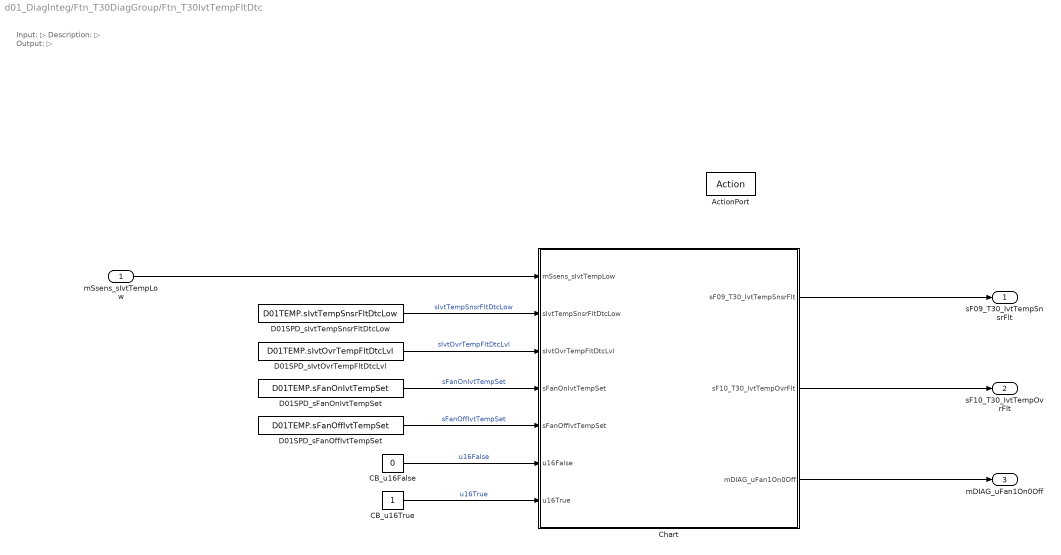
== system d01_Diaglnteg/Ftn_T30DiagGroup/Ftn_T30IvtTempFltDtc ==
  note: Input:
      | ▷
      | Description:
      | ▷
      | Output:
      | ▷
  mSsens_sIvtTempLow : Inport
  ActionPort : ActionPort  ActionPortLabel=case [ 18 ]:
  CB_u16False : Constant  Value=0  OutDataTypeStr=uint16
  CB_u16True : Constant  OutDataTypeStr=uint16
  Chart : Stateflow chart  TreatAsAtomicUnit=on
  D01SPD_sFanOffIvtTempSet : Constant  Value=D01TEMP.sFanOffIvtTempSet
  D01SPD_sFanOnIvtTempSet : Constant  Value=D01TEMP.sFanOnIvtTempSet
  D01SPD_sIvtOvrTempFltDtcLvl : Constant  Value=D01TEMP.sIvtOvrTempFltDtcLvl
  D01SPD_sIvtTempSnsrFltDtcLow : Constant  Value=D01TEMP.sIvtTempSnsrFltDtcLow
  sF09_T30_IvtTempSnsrFlt : Outport
  sF10_T30_IvtTempOvrFlt : Outport  Port=2
  mDIAG_uFan1On0Off : Outport  Port=3
  wires:
  mSsens_sIvtTempLow/1 -> Chart/1(mSsens_sIvtTempLow)
  Chart/1(sF09_T30_IvtTempSnsrFlt) -> sF09_T30_IvtTempSnsrFlt/1
  D01SPD_sIvtOvrTempFltDtcLvl/1 -> Chart/3(sIvtOvrTempFltDtcLvl)  "sIvtOvrTempFltDtcLvl"
  D01SPD_sFanOnIvtTempSet/1 -> Chart/4(sFanOnIvtTempSet)  "sFanOnIvtTempSet"
  D01SPD_sFanOffIvtTempSet/1 -> Chart/5(sFanOffIvtTempSet)  "sFanOffIvtTempSet"
  D01SPD_sIvtTempSnsrFltDtcLow/1 -> Chart/2(sIvtTempSnsrFltDtcLow)  "sIvtTempSnsrFltDtcLow"
  Chart/2(sF10_T30_IvtTempOvrFlt) -> sF10_T30_IvtTempOvrFlt/1
  CB_u16False/1 -> Chart/6(u16False)  "u16False"
  CB_u16True/1 -> Chart/7(u16True)  "u16True"
  Chart/3(mDIAG_uFan1On0Off) -> mDIAG_uFan1On0Off/1

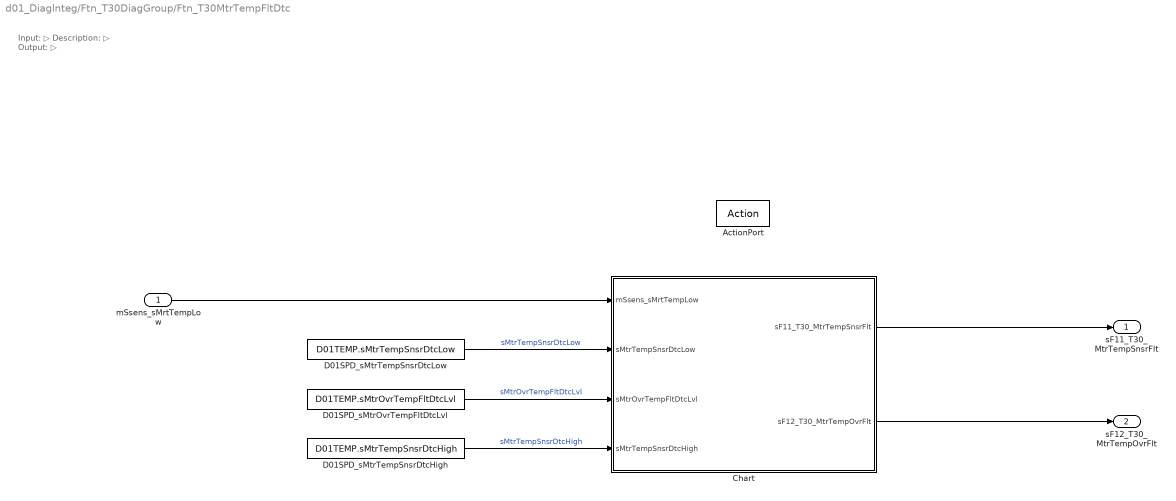
== system d01_Diaglnteg/Ftn_T30DiagGroup/Ftn_T30MtrTempFltDtc ==
  note: Input:
      | ▷
      | Description:
      | ▷
      | Output:
      | ▷
  mSsens_sMrtTempLow : Inport
  ActionPort : ActionPort  ActionPortLabel=case [ 24 ]:
  Chart : Stateflow chart  TreatAsAtomicUnit=on
  D01SPD_sMtrOvrTempFltDtcLvl : Constant  Value=D01TEMP.sMtrOvrTempFltDtcLvl
  D01SPD_sMtrTempSnsrDtcHigh : Constant  Value=D01TEMP.sMtrTempSnsrDtcHigh
  D01SPD_sMtrTempSnsrDtcLow : Constant  Value=D01TEMP.sMtrTempSnsrDtcLow
  sF11_T30_MtrTempSnsrFlt : Outport
  sF12_T30_MtrTempOvrFlt : Outport  Port=2
  wires:
  Chart/2(sF12_T30_MtrTempOvrFlt) -> sF12_T30_MtrTempOvrFlt/1
  D01SPD_sMtrTempSnsrDtcLow/1 -> Chart/2(sMtrTempSnsrDtcLow)  "sMtrTempSnsrDtcLow"
  D01SPD_sMtrTempSnsrDtcHigh/1 -> Chart/4(sMtrTempSnsrDtcHigh)  "sMtrTempSnsrDtcHigh"
  D01SPD_sMtrOvrTempFltDtcLvl/1 -> Chart/3(sMtrOvrTempFltDtcLvl)  "sMtrOvrTempFltDtcLvl"
  Chart/1(sF11_T30_MtrTempSnsrFlt) -> sF11_T30_MtrTempSnsrFlt/1
  mSsens_sMrtTempLow/1 -> Chart/1(mSsens_sMrtTempLow)

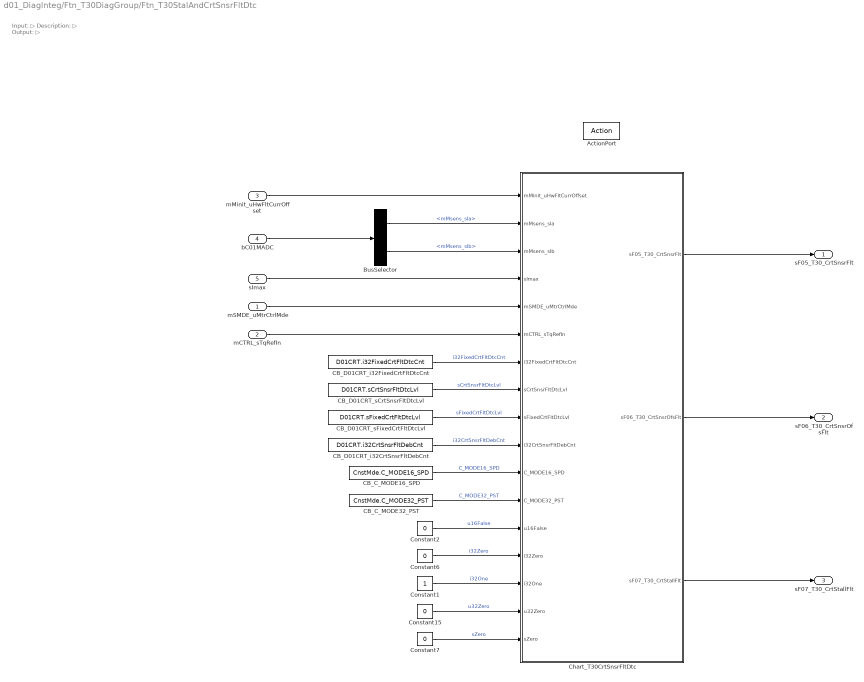
== system d01_Diaglnteg/Ftn_T30DiagGroup/Ftn_T30StalAndCrtSnsrFltDtc ==
  note: Input:
      | ▷
      | Description:
      | ▷
      | Output:
      | ▷
  mSMDE_uMtrCtrlMde : Inport
  mCTRL_sTqRefIn : Inport  Port=2
  mMinit_uHwFltCurrOffset : Inport  Port=3
  bC01MADC : Inport  Port=4
  sImax : Inport  Port=5  OutMin=0  OutMax=325.2
  ActionPort : ActionPort  ActionPortLabel=case [ 28 ]:
  BusSelector : BusSelector  OutputSignals=mMsens_sIa,mMsens_sIb
  CB_C_MODE16_SPD : Constant  Value=CnstMde.C_MODE16_SPD
  CB_C_MODE32_PST : Constant  Value=CnstMde.C_MODE32_PST
  CB_D01CRT_i32CrtSnsrFltDebCnt : Constant  Value=D01CRT.i32CrtSnsrFltDebCnt
  CB_D01CRT_i32FixedCrtFltDtcCnt : Constant  Value=D01CRT.i32FixedCrtFltDtcCnt
  CB_D01CRT_sCrtSnsrFltDtcLvl : Constant  Value=D01CRT.sCrtSnsrFltDtcLvl
  CB_D01CRT_sFixedCrtFltDtcLvl : Constant  Value=D01CRT.sFixedCrtFltDtcLvl
  Chart_T30CrtSnsrFltDtc : Stateflow chart  TreatAsAtomicUnit=on
  Constant1 : Constant  OutDataTypeStr=int32
  Constant15 : Constant  Value=0  OutDataTypeStr=uint32
  Constant2 : Constant  Value=0  OutDataTypeStr=uint16
  Constant6 : Constant  Value=0  OutDataTypeStr=int32
  Constant7 : Constant  Value=0  OutDataTypeStr=single
  sF05_T30_CrtSnsrFlt : Outport
  sF06_T30_CrtSnsrOfsFlt : Outport  Port=2  OutMin=0  OutMax=65536
  sF07_T30_CrtStallFlt : Outport  Port=3
  wires:
  CB_D01CRT_sCrtSnsrFltDtcLvl/1 -> Chart_T30CrtSnsrFltDtc/8(sCrtSnsrFltDtcLvl)  "sCrtSnsrFltDtcLvl"
  CB_D01CRT_i32FixedCrtFltDtcCnt/1 -> Chart_T30CrtSnsrFltDtc/7(i32FixedCrtFltDtcCnt)  "i32FixedCrtFltDtcCnt"
  sImax/1 -> Chart_T30CrtSnsrFltDtc/4(sImax)
  Constant15/1 -> Chart_T30CrtSnsrFltDtc/16(u32Zero)  "u32Zero"
  Constant1/1 -> Chart_T30CrtSnsrFltDtc/15(i32One)  "i32One"
  Chart_T30CrtSnsrFltDtc/2(sF06_T30_CrtSnsrOfsFlt) -> sF06_T30_CrtSnsrOfsFlt/1
  CB_D01CRT_i32CrtSnsrFltDebCnt/1 -> Chart_T30CrtSnsrFltDtc/10(i32CrtSnsrFltDebCnt)  "i32CrtSnsrFltDebCnt"
  Constant2/1 -> Chart_T30CrtSnsrFltDtc/13(u16False)  "u16False"
  Constant7/1 -> Chart_T30CrtSnsrFltDtc/17(sZero)  "sZero"
  Constant6/1 -> Chart_T30CrtSnsrFltDtc/14(i32Zero)  "i32Zero"
  mMinit_uHwFltCurrOffset/1 -> Chart_T30CrtSnsrFltDtc/1(mMinit_uHwFltCurrOffset)
  bC01MADC/1 -> BusSelector/1
  BusSelector/1 -> Chart_T30CrtSnsrFltDtc/2(mMsens_sIa)  "<mMsens_sIa>"
  BusSelector/2 -> Chart_T30CrtSnsrFltDtc/3(mMsens_sIb)  "<mMsens_sIb>"
  mSMDE_uMtrCtrlMde/1 -> Chart_T30CrtSnsrFltDtc/5(mSMDE_uMtrCtrlMde)
  mCTRL_sTqRefIn/1 -> Chart_T30CrtSnsrFltDtc/6(mCTRL_sTqRefIn)
  CB_C_MODE16_SPD/1 -> Chart_T30CrtSnsrFltDtc/11(C_MODE16_SPD)  "C_MODE16_SPD"
  CB_C_MODE32_PST/1 -> Chart_T30CrtSnsrFltDtc/12(C_MODE32_PST)  "C_MODE32_PST"
  CB_D01CRT_sFixedCrtFltDtcLvl/1 -> Chart_T30CrtSnsrFltDtc/9(sFixedCrtFltDtcLvl)  "sFixedCrtFltDtcLvl"
  Chart_T30CrtSnsrFltDtc/1(sF05_T30_CrtSnsrFlt) -> sF05_T30_CrtSnsrFlt/1
  Chart_T30CrtSnsrFltDtc/3(sF07_T30_CrtStallFlt) -> sF07_T30_CrtStallFlt/1

== stateflow chart d01_Diaglnteg/Ftn_T01DiagGroup/Ftn_T01HvdcFltDtc/Chart_T01HvdcFltDtc ==
  note: /********************************************************** Initial charging function ***************************************************/
      | 	if(Init_Charge == 1)
      | 	{
      | 		if(Vdc.low > DCLINK_DC_UNDER_WARN)								// 240
      | 		{
      | 			Init_Charge = 0;
      | 			DC_RELAY_ON;
      | 		}
      | 		else
      | 			DC_RELAY_OFF;
      | 	}
      | 	else
      | 	{
      | 		if(Vdc.low > DCLINK_DC_UNDER)									// 180
      | 		{
      | 			DC_RELAY_ON;
      | 			LED_AC_POWER_ON;
      | 		}
      | 		else
      | 		{
      | 			DC_RELAY_OFF;
      |
      | 			if(Vdc.low < 10)
      | 				LED_AC_POWER_OFF;
      | 			else
      | 				LED_AC_POWER_ON;
      | 		}
      | 	}
      | 	/****************************************************************************************************************************************/
  (default) -> (junction 60)
  (junction 60) -> (junction 65) [order 1] : [mMsens_sHVdcLow < sDcUdrVltFltDtcLvl]  /* < 180 [Vdc] */
  (junction 65) -> (junction 66) : {
      | sF04_T01_HvdcUdrVolFlt = Cnst_F04_HvdcUdrVolFlt;
      | mDIAG_uDcRly1ON0Off = u16False;
      | }
  (junction 60) -> (junction 22) [order 2] : {
      | mDIAG_uDcRly1ON0Off = u16True;
      | }
  (junction 22) -> (junction 23) [order 1] : [mMsens_sHVdcLow > sDcOvrVltFltDtcLvl]  /* > 405 [Vdc] */
  (junction 22) -> (junction 24) [order 2]
  (junction 23) -> (junction 31) : {
      | mDIAG_uChprOpr1On0Off = u16True;
      | uFlag_Hysteresis = u16True;
      | sF03_T01_HvdcOvrVolFlt = Cnst_F03_HvdcOvrVolFlt;
      | }
  (junction 24) -> (junction 25) [order 1] : [mMsens_sHVdcLow > sDcOvrWarnFltDtcLvl]  /* > 385 [Vdc] */
  (junction 24) -> (junction 26) [order 2]
  (junction 25) -> (junction 30) : {
      | mDIAG_uChprOpr1On0Off = u16True;
      | uFlag_Hysteresis = u16True;
      | }
  (junction 26) -> (junction 27) [order 1] : [mMsens_sHVdcLow > sDcOvrChpHysOprLvl]  /* > 375 [Vdc] */
  (junction 26) -> (junction 28) [order 2] : {
      | mDIAG_uChprOpr1On0Off = u16False;
      | sF04_T01_HvdcUdrVolFlt = u32False;
      | }
  (junction 27) -> (junction 47)
  (junction 47) -> (junction 49) [order 1] : [uFlag_Hysteresis == u16True]
  (junction 47) -> (junction 29) [order 2] : {
      | mDIAG_uChprOpr1On0Off = u16False;
      | }
  (junction 49) -> (junction 50) : {
      | mDIAG_uChprOpr1On0Off = u16True;
      | }
  (junction 29) -> (junction 28)
  (junction 50) -> (junction 29)
  (junction 30) -> (junction 50)
  (junction 31) -> (junction 30)
  (junction 66) -> (junction 31)
  (junction 28) -> (junction 32)
  data: mMsens_sHVdcLow input; sDcUdrVltFltDtcLvl input; sDcOvrChpHysOprLvl input; sDcOvrWarnFltDtcLvl input; sDcOvrVltFltDtcLvl input; mDIAG_uChprOpr1On0Off output uint16; mDIAG_uDcRly1ON0Off output uint16; u16False input; u16True input; uFlag_Hysteresis local uint16; Cnst_F03_HvdcOvrVolFlt constant uint32 =D02FLTS.F03_HvdcOvrVolFlt; sF03_T01_HvdcOvrVolFlt output uint32; sF04_T01_HvdcUdrVolFlt output uint32; Cnst_F04_HvdcUdrVolFlt constant uint32 =D02FLTS.F04_HvdcUdrVolFlt; u32False input

== stateflow chart d01_Diaglnteg/Ftn_T30DiagGroup/Ftn_T10MtrSpdFltDtc/Chart_T01Diag_OverCurrErrDtc ==
  (default) -> (junction 17)
  (junction 17) -> (junction 24) [order 1] : [mMTPST_sRpm >= sOvrSpdFltDtcLvl]
  (junction 17) -> (junction 27) [order 2] : {
      | mDIAG_i32CntCurrOver = i32Zero;
      | }
  (junction 24) -> (junction 37)
  (junction 37) -> (junction 16) [order 1] : [mDIAG_i32CntCurrOver >= i32OvrSpdFltDebCnt]
  (junction 37) -> (junction 33) [order 2] : {
      | mDIAG_i32CntCurrOver++;
      | }
  (junction 16) -> (junction 30) : {
      | mDIAG_i32CntCurrOver = i32OvrSpdFltDebCnt;
      | sF13_T10_MtrSpdFlt =  Cnst_F13_MtrSpdFlt;
      | }
  (junction 33) -> (junction 27)
  (junction 30) -> (junction 33)
  (junction 27) -> (junction 460)
  data: mMTPST_sRpm input; i32OvrSpdFltDebCnt input; sOvrSpdFltDtcLvl input; sF13_T10_MtrSpdFlt output uint32; mDIAG_i32CntCurrOver output int32; Cnst_F13_MtrSpdFlt constant uint32 =D02FLTS.F13_MtrSpdFlt; i32Zero input

== stateflow chart d01_Diaglnteg/Ftn_T01DiagGroup/Ftn_T01GateAndEstpFltDtc/Chart_T01GateAndEstpFltDtc ==
  (default) -> (junction 12)
  (junction 12) -> (junction 13) [order 1] : [mBSW_uGateFltDtc == u16False]
  (junction 12) -> (junction 14) [order 2] : /* No Action */
  (junction 13) -> (junction 15) : {
      | sF02_T01_IgptShrtFlt = Cnst_F02_IgptShrtFlt;
      | }
  (junction 15) -> (junction 14)
  (junction 14) -> (junction 24)
  (junction 24) -> (junction 21) [order 1] : [mCRX_uEmg == u16False]
  (junction 24) -> (junction 26) [order 2] : /* No Action */
  (junction 21) -> (junction 25) : {
      | sF01_T01_EstopSwitchFlt = Cnst_F01_EstopSwitchFlt;
      | }
  (junction 25) -> (junction 26)
  (junction 26) -> (junction 40)
  data: mCRX_uEmg input; mBSW_uGateFltDtc input; u16False input; sF01_T01_EstopSwitchFlt output uint32; sF02_T01_IgptShrtFlt output uint32; Cnst_F01_EstopSwitchFlt constant uint32 =D02FLTS.F01_EstopSwitchFlt; Cnst_F02_IgptShrtFlt constant uint32 =D02FLTS.F02_IgptShrtFlt

== stateflow chart d01_Diaglnteg/Ftn_T30DiagGroup/Ftn_T30IvtTempFltDtc/Chart ==
  (default) -> (junction 17)
  (junction 17) -> (junction 18) [order 1] : [mSsens_sIvtTempLow > sIvtOvrTempFltDtcLvl]
  (junction 17) -> (junction 29) [order 2]
  (junction 18) -> (junction 20) : {
      | sF10_T30_IvtTempOvrFlt = Cnst_F010_IvtTempOvrFlt;
      | }
  (junction 29) -> (junction 31) [order 1] : [mSsens_sIvtTempLow > sFanOnIvtTempSet]
  (junction 31) -> (junction 32) : {
      | mDIAG_uFan1On0Off = u16True;
      | }
  (junction 29) -> (junction 39) [order 2]
  (junction 39) -> (junction 41) [order 1] : [mSsens_sIvtTempLow < sFanOffIvtTempSet]
  (junction 39) -> (junction 22) [order 2]
  (junction 41) -> (junction 37) : {
      | mDIAG_uFan1On0Off = u16False;
      | }
  (junction 22) -> (junction 26) [order 1] : [mSsens_sIvtTempLow <sIvtTempSnsrFltDtcLow]
  (junction 22) -> (junction 19) [order 2] : /* No Action */
  (junction 26) -> (junction 24) : {
      | sF09_T30_IvtTempSnsrFlt = Cnst_F09_IvtTempSnsrFlt;
      | }
  (junction 24) -> (junction 19)
  (junction 37) -> (junction 24)
  (junction 32) -> (junction 37)
  (junction 20) -> (junction 32)
  (junction 19) -> (junction 21)
  data: sF09_T30_IvtTempSnsrFlt output uint32; sF10_T30_IvtTempOvrFlt output uint32; mSsens_sIvtTempLow input; sIvtTempSnsrFltDtcLow input; sIvtOvrTempFltDtcLvl input; sFanOnIvtTempSet input; sFanOffIvtTempSet input; u16False input; Cnst_F09_IvtTempSnsrFlt constant uint32 =D02FLTS.F09_IvtTempSnsrFlt; Cnst_F010_IvtTempOvrFlt constant uint32 =D02FLTS.F010_IvtTempOvrFlt; mDIAG_uFan1On0Off output uint16; u16True input

== stateflow chart d01_Diaglnteg/Ftn_T30DiagGroup/Ftn_T30MtrTempFltDtc/Chart ==
  (default) -> (junction 17)
  (junction 17) -> (junction 18) [order 1] : [(mSsens_sMrtTempLow < sMtrTempSnsrDtcLow)||(mSsens_sMrtTempLow > sMtrTempSnsrDtcHigh)]
  (junction 17) -> (junction 29) [order 2]
  (junction 18) -> (junction 20) : {
      | sF11_T30_MtrTempSnsrFlt = Cnst_F11_MtrTempSnsrFlt;
      | }
  (junction 29) -> (junction 31) [order 1] : [mSsens_sMrtTempLow >  sMtrOvrTempFltDtcLvl]
  (junction 29) -> (junction 19) [order 2] : /* No Action */
  (junction 31) -> (junction 32) : {
      | sF12_T30_MtrTempOvrFlt = Cnst_F12_MtrTempOvrFlt;
      | }
  (junction 32) -> (junction 19)
  (junction 20) -> (junction 32)
  (junction 19) -> (junction 21)
  data: sF11_T30_MtrTempSnsrFlt output uint32; sF12_T30_MtrTempOvrFlt output uint32; mSsens_sMrtTempLow input; sMtrTempSnsrDtcLow input; sMtrOvrTempFltDtcLvl input; sMtrTempSnsrDtcHigh input; Cnst_F12_MtrTempOvrFlt constant uint32 =D02FLTS.F12_MtrTempOvrFlt; Cnst_F11_MtrTempSnsrFlt constant uint32 =D02FLTS.F11_MtrTempSnsrFlt

== stateflow chart d01_Diaglnteg/Ftn_T30DiagGroup/Ftn_T30StalAndCrtSnsrFltDtc/Chart_T30CrtSnsrFltDtc ==
  note: a상 고정
  note: b상 고정
  (default) -> (junction 83)
  (junction 83) -> (junction 80) [order 1] : [mMinit_uHwFltCurrOffset ~= u16False]
  (junction 83) -> (junction 199) [order 2]
  (junction 80) -> (junction 77) : {
      | sF06_T30_CrtSnsrOfsFlt = Cnst_F06_CrtSnsrOfsFlt;
      | }
  (junction 199) -> (junction 239) [order 1] : [sImax >= sCrtSnsrFltDtcLvl]
  (junction 199) -> (junction 210) [order 2] : {
      | i32CntSnsrFlt = i32Zero;
      | }
  (junction 239) -> (junction 240)
  (junction 240) -> (junction 201) [order 1] : [i32CntSnsrFlt >= i32CrtSnsrFltDebCnt]
  (junction 240) -> (junction 244) [order 2] : {
      | i32CntSnsrFlt++;
      | }
  (junction 201) -> (junction 208) : {
      | i32CntSnsrFlt = i32CrtSnsrFltDebCnt;
      | sF05_T30_CrtSnsrFlt = Cnst_F05_CrtSnsrFlt;
      | }
  (junction 244) -> (junction 210)
  (junction 208) -> (junction 244)
  (junction 77) -> (junction 208)
  (junction 210) -> (junction 256)
  (junction 256) -> (junction 257) [order 1] : [sF07_T30_CrtStallFlt == u32Zero]
  (junction 256) -> (junction 164) [order 2] : {
      | i32CntIaFixedCurrUp = i32Zero;
      | i32CntIaFixedCurrDown = i32Zero;
      | i32CntIbFixedCurrUp = i32Zero;
      | i32CntIbFixedCurrDown = i32Zero;
      | }
  (junction 257) -> (junction 130)
  (junction 130) -> (junction 131) [order 1] : [((mSMDE_uMtrCtrlMde ==C_MODE16_SPD)||(mSMDE_uMtrCtrlMde == C_MODE32_PST))&&(mCTRL_sTqRefIn >= sFixedCrtFltDtcLvl)]
  (junction 130) -> (junction 139) [order 2] : {
      | i32CntIaFixedCurrUp = i32Zero;
      | i32CntIaFixedCurrDown = i32Zero;
      | i32CntIbFixedCurrUp = i32Zero;
      | i32CntIbFixedCurrDown = i32Zero;
      | }
  (junction 131) -> (junction 143)
  (junction 143) -> (junction 146) [order 1] : [mMsens_sIa > sZero]
  (junction 143) -> (junction 150) [order 2] : {
      | i32CntIaFixedCurrDown = i32CntIaFixedCurrDown + i32One;
      | i32CntIaFixedCurrUp = i32Zero;
      | }
  (junction 146) -> (junction 148) : {
      | i32CntIaFixedCurrUp = i32CntIaFixedCurrUp + i32One;
      | i32CntIaFixedCurrDown = i32Zero;
      | }
  (junction 148) -> (junction 150)
  (junction 150) -> (junction 170)
  (junction 170) -> (junction 173) [order 1] : [(i32CntIaFixedCurrUp + i32CntIaFixedCurrDown) > i32FixedCrtFltDtcCnt]
  (junction 170) -> (junction 177) [order 2] : /* No action */
  (junction 173) -> (junction 175) : {
      | sF07_T30_CrtStallFlt = Cnst_F07_CrtStallFlt;
      | }
  (junction 175) -> (junction 177)
  (junction 177) -> (junction 296)
  (junction 296) -> (junction 301) [order 1] : [mMsens_sIb > sZero]
  (junction 296) -> (junction 315) [order 2] : {
      | i32CntIbFixedCurrDown = i32CntIbFixedCurrDown + i32One;
      | i32CntIbFixedCurrUp = i32Zero;
      | }
  (junction 301) -> (junction 306) : {
      | i32CntIbFixedCurrUp = i32CntIbFixedCurrUp + i32One;
      | i32CntIbFixedCurrDown = i32Zero;
      | }
  (junction 306) -> (junction 315)
  (junction 315) -> (junction 304)
  (junction 304) -> (junction 308) [order 1] : [(i32CntIbFixedCurrUp + i32CntIbFixedCurrDown) > i32FixedCrtFltDtcCnt]
  (junction 304) -> (junction 298) [order 2] : /* No action */
  (junction 308) -> (junction 314) : {
      | sF07_T30_CrtStallFlt = Cnst_F07_CrtStallFlt;
      | }
  (junction 139) -> (junction 164)
  (junction 298) -> (junction 139)
  (junction 314) -> (junction 298)
  (junction 164) -> (junction 302)
  data: sF05_T30_CrtSnsrFlt output uint32; mMinit_uHwFltCurrOffset input; mMsens_sIa input; mMsens_sIb input; sImax input; mSMDE_uMtrCtrlMde input; mCTRL_sTqRefIn input; i32FixedCrtFltDtcCnt input; sCrtSnsrFltDtcLvl input; sFixedCrtFltDtcLvl input; i32CrtSnsrFltDebCnt input; C_MODE16_SPD input; C_MODE32_PST input; sF06_T30_CrtSnsrOfsFlt output uint32; Cnst_F06_CrtSnsrOfsFlt constant uint32 =D02FLTS.F06_CrtSnsrOfsFlt; u16False input; i32CntIaFixedCurrUp local int32; i32CntIaFixedCurrDown local int32; i32CntSnsrFlt local int32; i32Zero input; i32One input; u32Zero input; sZero input; i32CntIbFixedCurrDown local int32; i32CntIbFixedCurrUp local int32; Cnst_F05_CrtSnsrFlt constant uint32 =D02FLTS.F05_CrtSnsrFlt; sF07_T30_CrtStallFlt output uint32; Cnst_F07_CrtStallFlt constant uint32 =D02FLTS.F07_CrtStallFlt

== stateflow chart d01_Diaglnteg/Ftn_T01Diaglntegration/Ftn_FaultIntegration ==
  (default) -> (junction 559)
  (junction 559) -> (junction 563) : {
      | u32FltSum = uint32(sF01_T01_EstopSwitchFlt|sF02_T01_IgptShrtFlt|sF03_T01_HvdcOvrVolFlt|sF04_T01_HvdcUdrVolFlt|sF05_T30_CrtSnsrFlt|...
      | sF06_T30_CrtSnsrOfsFlt|sF07_T30_CrtStallFlt|sF08_T01_CrtOvrFlt|sF09_T30_IvtTempSnsrFlt|sF10_T30_IvtTempOvrFlt|...
      | sF11_T30_MtrTempSnsrFlt|sF12_T30_MtrTempOvrFlt|sF13_T10_MtrSpdFlt|F16_T10_InitNvRam);
      | }
  (junction 563) -> (junction 561) : {
      | u32FltSum = uint32(u32FltSum & u32DisFltAll);
      | }
  (junction 561) -> (junction 571) [order 1] : [u32FltSum ~= u32Zero]
  (junction 561) -> (junction 567) [order 2] : {
      | mDIAG_uFltStat = u16False;
      | F00 = u32Zero;
      | }
  (junction 571) -> (junction 572) : {
      | mDIAG_uFltStat = u16True;
      | F00 = Cnst_sF00;
      | }
  (junction 572) -> (junction 567)
  (junction 567) -> (junction 568) : {
      | mDIAG_u32FltAll = uint32(F00|u32FltSum);
      | }
  data: sF01_T01_EstopSwitchFlt input; sF02_T01_IgptShrtFlt input; sF03_T01_HvdcOvrVolFlt input; sF04_T01_HvdcUdrVolFlt input; sF05_T30_CrtSnsrFlt input; sF06_T30_CrtSnsrOfsFlt input; sF07_T30_CrtStallFlt input; sF08_T01_CrtOvrFlt input; sF09_T30_IvtTempSnsrFlt input; sF10_T30_IvtTempOvrFlt input; sF11_T30_MtrTempSnsrFlt input; sF12_T30_MtrTempOvrFlt input; sF13_T10_MtrSpdFlt input; F16_T10_InitNvRam input; mDIAG_uFltStat output uint16; mDIAG_u32FltAll output uint32; u32DisFltAll input; u32FltSum local uint32; Cnst_sF00 constant uint32 =1; F00 local double; u16False input; u16True input; u32Zero input

== stateflow chart d01_Diaglnteg/Ftn_T30DiagGroup/Ftn_T30InitNvRamDtc/Chart_T30InitNvRamDtc ==
  (default) -> (junction 23)
  (junction 23) -> (junction 30) [order 1] : [mBSW_uInitNvRam == u16True]
  (junction 23) -> (junction 31) [order 2] : /* No Action */
  (junction 30) -> (junction 32) : {
      | sF16_T10_InitNvRam = Cnst_F16_T10_InitNvRam;
      | }
  (junction 32) -> (junction 31)
  (junction 31) -> (junction 33)
  data: mBSW_uInitNvRam input; u16True input; sF16_T10_InitNvRam output uint32; Cnst_F16_T10_InitNvRam constant uint32 =D02FLTS.F16_InitNvRam

== stateflow chart d01_Diaglnteg/Ftn_T01DiagGroup/Ftn_T01CrtFltDtc/Chart_T01Diag_OverCurrErrDtc ==
  (default) -> (junction 17)
  (junction 17) -> (junction 24) [order 1] : [sImax >= sOvrCrtFltDtcLvl]
  (junction 17) -> (junction 27) [order 2] : {
      | mDIAG_i32CntCrOvr = i32Zero;
      | }
  (junction 24) -> (junction 37)
  (junction 37) -> (junction 16) [order 1] : [mDIAG_i32CntCrOvr >= i32CrtFltDebCnt]
  (junction 37) -> (junction 33) [order 2] : {
      | mDIAG_i32CntCrOvr++;
      | }
  (junction 16) -> (junction 30) : {
      | mDIAG_i32CntCrOvr = i32CrtFltDebCnt;
      | sF08_T01_CrtOvrFlt =  Cnst_F08_CrtOvrFlt;
      | }
  (junction 33) -> (junction 27)
  (junction 30) -> (junction 33)
  (junction 27) -> (junction 460)
  data: sImax input; mDIAG_i32CntCrOvr output int32; i32CrtFltDebCnt input; sOvrCrtFltDtcLvl input; sF08_T01_CrtOvrFlt output uint32; Cnst_F08_CrtOvrFlt constant uint32 =D02FLTS.F08_CrtOvrFlt; i32Zero input
